simulink model "ejh62b"  (Simulink 3.00)
settings: Solver=ode45  StartTime=0.0  StopTime=10.0  RelTol=1e-3
libraries: HEMERO x1
settings Model: LastModifiedBy=Administrador

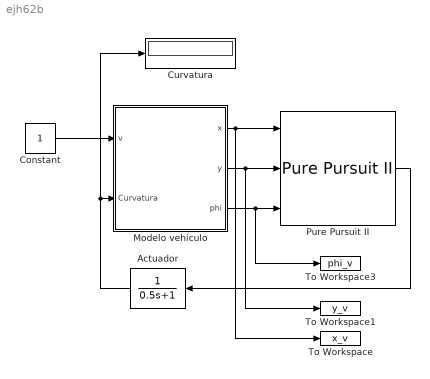
== system ejh62b ==
  Actuador : TransferFcn  Orientation=left  Numerator=[1]  Denominator=[0.5 1]
  Constant : Constant  Value=1
  Curvatura : Display
      settings: Format=short
  Modelo vehículo : Subsystem  mask{x_inicial=0, y_inicial=0.5, phi_inicial=0}
      mask prompts: x_inicial "Valor inicial de la coordenada x:"; y_inicial "Valor inicial de la coordenada y:"; phi_inicial "Valor inicial de la orientación:"
  Pure Pursuit II : HEMERO/Robots móviles/Control de robots móviles/Métodos geométricos/Pure Pursuit II  x_camino=x  y_camino=y  s=s
  To Workspace : ToWorkspace  VariableName=x_v  SampleTime=-1  SaveFormat=Matrix
  To Workspace1 : ToWorkspace  VariableName=y_v  SampleTime=-1  SaveFormat=Matrix
  To Workspace3 : ToWorkspace  VariableName=phi_v  SampleTime=-1  SaveFormat=Matrix
  wires:
  Constant/1 -> Modelo vehículo/1(v)
  Actuador/1 -> Modelo vehículo/2(Curvatura), Curvatura/1
  Modelo vehículo/1(x) -> Pure Pursuit II/1, To Workspace/1
  Modelo vehículo/2(y) -> Pure Pursuit II/2, To Workspace1/1
  Modelo vehículo/3(phi) -> Pure Pursuit II/3, To Workspace3/1
  Pure Pursuit II/1 -> Actuador/1

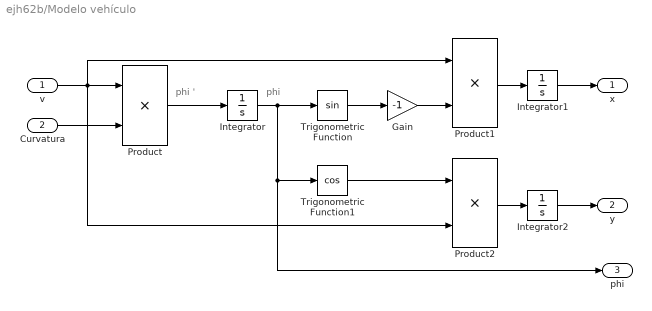
== system ejh62b/Modelo vehículo ==
  note: phi '
  note: phi
  v : Inport  Port=1  PortWidth=-1  SampleTime=-1  DataType=auto
      settings: SignalType=auto
  Curvatura : Inport  Port=2  PortWidth=-1  SampleTime=-1  DataType=auto
      settings: SignalType=auto
  Gain : Gain  Gain=-1  SaturateOnIntegerOverflow=on
  Integrator : Integrator  ExternalReset=none  InitialConditionSource=internal  InitialCondition=phi_inicial  LimitOutput=off  UpperSaturationLimit=inf  LowerSaturationLimit=-inf  ShowSaturationPort=off  ShowStatePort=off  AbsoluteTolerance=auto
  Integrator1 : Integrator  ExternalReset=none  InitialConditionSource=internal  InitialCondition=x_inicial  LimitOutput=off  UpperSaturationLimit=inf  LowerSaturationLimit=-inf  ShowSaturationPort=off  ShowStatePort=off  AbsoluteTolerance=auto
  Integrator2 : Integrator  ExternalReset=none  InitialConditionSource=internal  InitialCondition=y_inicial  LimitOutput=off  UpperSaturationLimit=inf  LowerSaturationLimit=-inf  ShowSaturationPort=off  ShowStatePort=off  AbsoluteTolerance=auto
  Product : Product  Inputs=2  SaturateOnIntegerOverflow=on
  Product1 : Product  Inputs=2  SaturateOnIntegerOverflow=on
  Product2 : Product  Inputs=2  SaturateOnIntegerOverflow=on
  Trigonometric Function : Trigonometry  Operator=sin  OutputSignalType=auto
  Trigonometric Function1 : Trigonometry  Operator=cos  OutputSignalType=auto
  x : Outport  Port=1
  y : Outport  Port=2
  phi : Outport  Port=3
  wires:
  Curvatura/1 -> Product/2
  Product/1 -> Integrator/1
  Integrator/1 -> Trigonometric Function/1, Trigonometric Function1/1, phi/1
  Trigonometric Function/1 -> Gain/1
  Gain/1 -> Product1/2
  v/1 -> Product/1, Product1/1, Product2/2
  Trigonometric Function1/1 -> Product2/1
  Product1/1 -> Integrator1/1
  Product2/1 -> Integrator2/1
  Integrator2/1 -> y/1
  Integrator1/1 -> x/1
